simulink library "Driver_Long_Lateral"  (R2025a)
settings: Solver=VariableStepAuto  StartTime=0.0  StopTime=10.0  RelTol=1e-3
undefined symbols (not defined in the file): Driver, Vehicle
libraries: Maneuver_Get_Pose x1
Description:
  | Simscape Vehicle Templates Library
  | 
  | Copyright 2018-2025 The MathWorks, Inc.
settings Model: Creator=smiller  LastModifiedBy=smiller
settings SolverCC: AlgebraicLoopSolver=TrustRegion
settings DataIOCC: ReturnWorkspaceOutputs=off
settings DebuggingCC: UnconnectedInputMsg=warning  UnconnectedOutputMsg=warning  UnconnectedLineMsg=warning  ArithmeticOperatorsInVariantConditions=warning
settings ModelReferenceCC: EnableRefExpFcnMdlSchedulingChecks=on
settings SFSimCC: CustomCodeUndefinedFunction=UseInterfaceOnly
settings RTWCC: GPUComputeCapability=3.5  DLArmComputeVersion=19.05

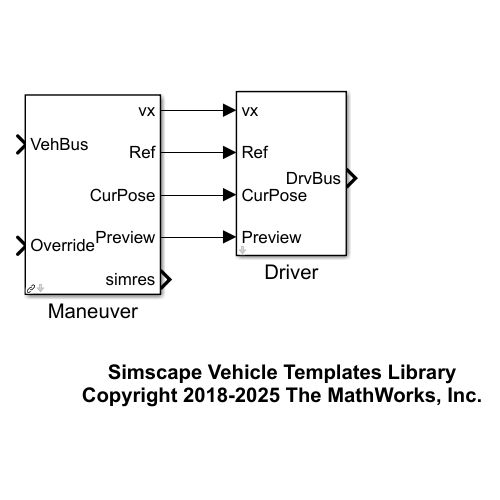
[thumbnail: Simulink's stored preview of the top-level diagram]
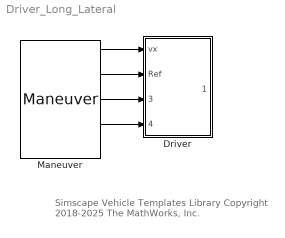
== system Driver_Long_Lateral ==
  note: Simscape Vehicle Templates Library
      | Copyright 2018-2025 The MathWorks, Inc.
  Driver : Subsystem  mask(Driver Behavior){Driver=Driver}
      mask help: Models driver behavior to follow prescribed vehicle trajectory, including path and speed.
  Maneuver : Maneuver_Get_Pose/Maneuver  Maneuver=Maneuver  popup_window=No
  wires:
  Maneuver/1 -> Driver/1(vx)
  Maneuver/2 -> Driver/2(Ref)
  Maneuver/3 -> Driver/3(CurPose)
  Maneuver/4 -> Driver/4(Preview)

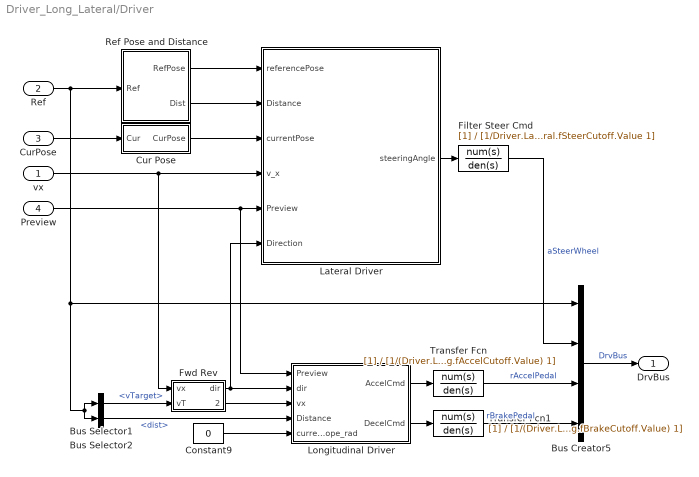
== system Driver_Long_Lateral/Driver ==
  vx : Inport
  Ref : Inport  Port=2
  CurPose : Inport  Port=3
  Preview : Inport  Port=4
  Bus Creator5 : BusCreator  Inputs=4
  Bus Selector1 : BusSelector  OutputSignals=vTarget
  Bus Selector2 : BusSelector  OutputSignals=dist
  Constant9 : Constant  Value=0
  Cur Pose : Subsystem
  Filter Steer Cmd : TransferFcn  Denominator=[1/Driver.Lateral.fSteerCutoff.Value 1]
  Fwd Rev : Subsystem
  Lateral Driver : Subsystem  Variant=on  VariantControlMode=label  VariantControl=Choice  LabelModeActiveChoice=Stanley  mask{Lateral=Driver.Lateral, VariantLabel=Driver.Lateral.class.Value}
      mask prompts: Lateral "Lateral Driver Parameters (structure)"; VariantLabel "Variant Label"
      mask init:
      | curblk = gcb;
      | 
      | % Set variant for this block 
      | set_param(curblk,'LabelModeActiveChoice',VariantLabel);
  Longitudinal Driver : Subsystem  mask(Longitudinal Driver (Velocity-tracking Controller)){SPEED_LOOKAHEAD_TIME=Driver.Long.FFLookahead.Value, C_ROLLING_RESISTANCE_COEFF=Driver.Long.NRollingResistance.Value, ROAD_FRICTION_COEFF=Driver.Long.NRoadFriction.Value, mVehicle=Driver.Long.mVehicle.Value, gGravity=Driver.Long.gGravity.Value, FTractive=Driver.Long.FTractive.Value, KP_SPEED=Driver.Long.Kp.Value, KI_SPEED=Driver.Long.Ki.Value, MAX_ACCEL_MPS2=Driver.Long.gMaxAccel.Value, MAX_DECEL_MPS2=Driver.Long.gMaxDecel.Value, Cdrag=Vehicle.Chassis.Aero.CD.Value, rho_air=Vehicle.Chassis.Aero.rho_air.Value, ARef=Vehicle.Chassis.Aero.ARef.Value}
      mask prompts: SPEED_LOOKAHEAD_TIME "Lookahead time (s)"; C_ROLLING_RESISTANCE_COEFF "Rolling resistance coefficient"; ROAD_FRICTION_COEFF "Road friction coefficient"; mVehicle "Total Vehicle mass (kg)"; gGravity "Gravity (m/s)"; FTractive "Tractive Force (N)"; KP_SPEED "Proportional gain, Kp"; KI_SPEED "Integral gain, Ki"; MAX_ACCEL_MPS2 "Max acceleration (m/s^2, positive number))"; MAX_DECEL_MPS2 "Max deceleration (m/s^2, must be negative)"; Cdrag "Drag coefficient"; rho_air "Density of air (kg/m^3)"; ARef "Frontal Area (m^2)"
      mask help: Implements a PI controller with feedforward for velocity tracking.
      mask DialogControl cont_feedforward Prompt: Feed-Forward Controller parameters
      mask DialogControl cont_feedback Prompt: Feedback Controller parameters
      mask DialogControl cont_drag Prompt: Drag
  Ref Pose and Distance : Subsystem
  Transfer Fcn : TransferFcn  Denominator=[1/(Driver.Long.fAccelCutoff.Value) 1]
  Transfer Fcn1 : TransferFcn  Denominator=[1/(Driver.Long.fBrakeCutoff.Value) 1]
  DrvBus : Outport  VectorParamsAs1DForOutWhenUnconnected=off
  wires:
  Filter Steer Cmd/1 -> Bus Creator5/2  "aSteerWheel"
  Ref Pose and Distance/1(RefPose) -> Lateral Driver/1(referencePose)
  Ref/1 -> Ref Pose and Distance/1(Ref), Bus Selector1/1, Bus Selector2/1, Bus Creator5/1
  Transfer Fcn/1 -> Bus Creator5/3  "rAccelPedal"
  Transfer Fcn1/1 -> Bus Creator5/4  "rBrakePedal"
  Longitudinal Driver/2(DecelCmd) -> Transfer Fcn1/1
  Longitudinal Driver/1(AccelCmd) -> Transfer Fcn/1
  Bus Creator5/1 -> DrvBus/1  "DrvBus"
  Constant9/1 -> Longitudinal Driver/5(current_slope_rad)
  CurPose/1 -> Cur Pose/1(Cur)
  Cur Pose/1(CurPose) -> Lateral Driver/3(currentPose)
  vx/1 -> Lateral Driver/4(v_x), Fwd Rev/1(vx)
  Fwd Rev/1(dir) -> Lateral Driver/6(Direction), Longitudinal Driver/2(dir)
  Lateral Driver/1(steeringAngle) -> Filter Steer Cmd/1
  Preview/1 -> Lateral Driver/5(Preview), Longitudinal Driver/1(Preview)
  Ref Pose and Distance/2(Dist) -> Lateral Driver/2(Distance)
  Bus Selector1/1 -> Fwd Rev/2(vT)  "<vTarget>"
  Fwd Rev/2(vxFwRv) -> Longitudinal Driver/3(vx)
  Bus Selector2/1 -> Longitudinal Driver/4(Distance)  "<dist>"

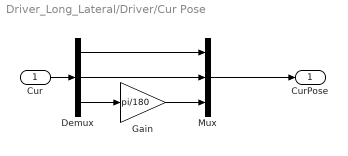
== system Driver_Long_Lateral/Driver/Cur Pose ==
  Cur : Inport
  Demux : Demux  Outputs=3
  Gain : Gain  Gain=pi/180
  Mux : Mux  Inputs=3
  CurPose : Outport  VectorParamsAs1DForOutWhenUnconnected=off
  wires:
  Demux/1 -> Mux/1
  Cur/1 -> Demux/1
  Mux/1 -> CurPose/1
  Demux/2 -> Mux/2
  Demux/3 -> Gain/1
  Gain/1 -> Mux/3

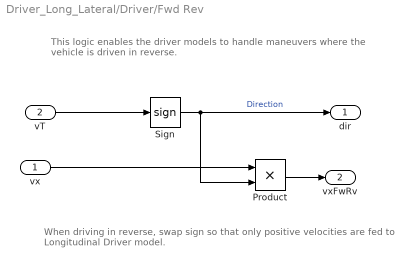
== system Driver_Long_Lateral/Driver/Fwd Rev ==
  note: When driving in reverse, swap sign so that only positive velocities are fed to Longitudinal Driver model.
  note: This logic enables the driver models to handle maneuvers where the vehicle is driven in reverse.
  vx : Inport
  vT : Inport  Port=2
  Product : Product
  Sign : Signum  ZeroCross=off
  dir : Outport
  vxFwRv : Outport  Port=2
  wires:
  vT/1 -> Sign/1
  Sign/1 -> dir/1, Product/2  "Direction"
  vx/1 -> Product/1
  Product/1 -> vxFwRv/1

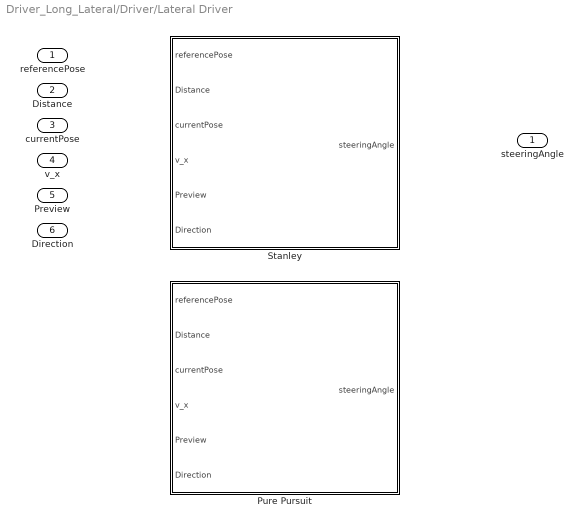
== system Driver_Long_Lateral/Driver/Lateral Driver ==
  referencePose : Inport
  Distance : Inport  Port=2
  currentPose : Inport  Port=3
  v_x : Inport  Port=4
  Preview : Inport  Port=5
  Direction : Inport  Port=6
  Pure Pursuit : Subsystem  VariantControl=Pure_Pursuit  mask(Lateral Driver (Pure Pursuit)){MAX_STEERING_ANGLE_DEG=Lateral.aMaxSteer.Value, L_AXLE_DIST=Lateral.xWheelbase.Value, LOOKAHEAD_GAIN_KPP=Lateral.Pursuit.kLookahead.Value, MIN_LOOKAHEAD_DIST=Lateral.Pursuit.xLookaheadMin.Value, MAX_LOOKAHEAD_DIST=Lateral.Pursuit.xLookaheadMax.Value, HEADING_WEIGHT_KH=Lateral.Pursuit.nWeightHeadingErr.Value}
      mask prompts: MAX_STEERING_ANGLE_DEG "Maximum steering angle (degrees)"; L_AXLE_DIST "Distance from the vehicle's reference point (currentPose) to the front axle (m)"; LOOKAHEAD_GAIN_KPP "Proportional gain for lookahead distance (Ld = K_pp * v_x)"; MIN_LOOKAHEAD_DIST "Minimum lookahead distance (m)"; MAX_LOOKAHEAD_DIST "Maximum lookahead distance (m)"; HEADING_WEIGHT_KH "Weight for the heading error term"
      mask help:
      | Implements PurePursuit method for lateral control.
      | Supports forward and reverse driving.
      | Pure Pursuit is based on Coulter, R. Craig. (1992). Implementation of the Pure Pursuit Path Tracking Algorithm. Carnegie Mellon University, The Robotics Institute. Technical Report CMU-RI-TR-92-01.
      mask DialogControl Container5 Prompt: Vehicle Parameters
      mask DialogControl Container4 Prompt: Pure Pursuit Method Parameters
  Stanley : Subsystem  VariantControl=Stanley  mask(Lateral Driver (Stanley)){MAX_STEERING_ANGLE_DEG=Lateral.aMaxSteer.Value, L_AXLE_DIST=Lateral.xWheelbase.Value, K_cte_forward=Lateral.Stanley.NForward.Value, K_cte_reverse=Lateral.Stanley.NReverse.Value}
      mask prompts: MAX_STEERING_ANGLE_DEG "Maximum steering angle (degrees)"; L_AXLE_DIST "Distance from the vehicle's reference point (currentPose) to the front axle (m)"; K_cte_forward "Cross-track error gain for forward"; K_cte_reverse "Cross-track error gain for reverse"
      mask help:
      | Implements Stanley method for lateral control.
      | Supports forward and reverse driving.
      | Stanley method is based on Hoffmann et al. (2007), "Autonomous Automobile Trajectory Tracking for Off-Road Driving"
      mask DialogControl Container5 Prompt: Vehicle Parameters
      mask DialogControl Container3 Prompt: Stanley Method Parameters
  steeringAngle : Outport

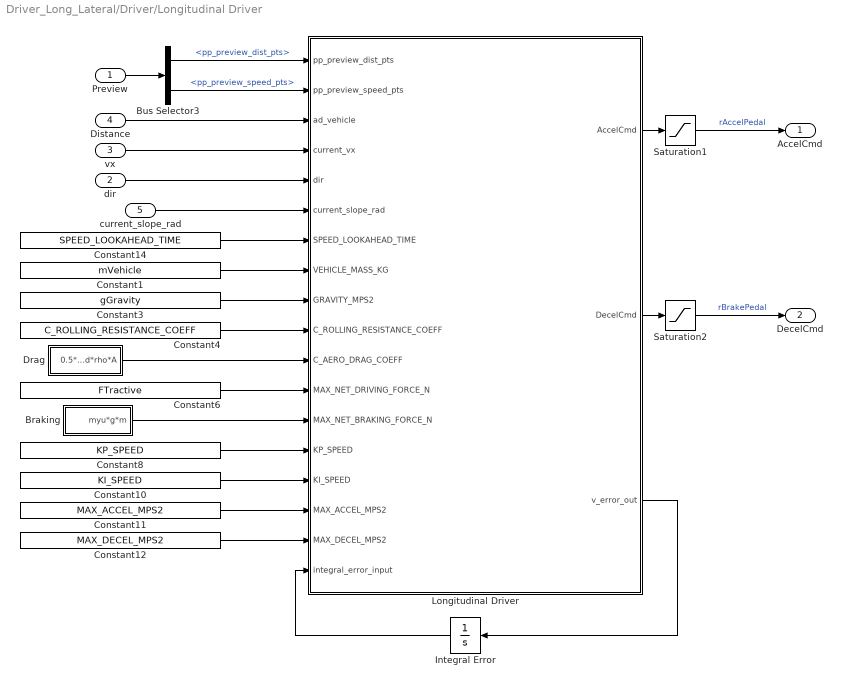
== system Driver_Long_Lateral/Driver/Longitudinal Driver ==
  Preview : Inport
  dir : Inport  Port=2
  vx : Inport  Port=3
  Distance : Inport  Port=4
  current_slope_rad : Inport  Port=5
  Braking : Subsystem
  Bus Selector3 : BusSelector  OutputSignals=pp_preview_dist_pts,pp_preview_speed_pts
  Constant1 : Constant  Value=mVehicle
  Constant10 : Constant  Value=KI_SPEED
  Constant11 : Constant  Value=MAX_ACCEL_MPS2
  Constant12 : Constant  Value=MAX_DECEL_MPS2
  Constant14 : Constant  Value=SPEED_LOOKAHEAD_TIME
  Constant3 : Constant  Value=gGravity
  Constant4 : Constant  Value=C_ROLLING_RESISTANCE_COEFF
  Constant6 : Constant  Value=FTractive
  Constant8 : Constant  Value=KP_SPEED
  Drag : Subsystem
  Integral Error : Integrator
  Longitudinal Driver : MATLAB Function  TreatAsAtomicUnit=on
  Saturation1 : Saturate  UpperLimit=1  LowerLimit=0  ZeroCross=off
  Saturation2 : Saturate  UpperLimit=1  LowerLimit=0  ZeroCross=off
  AccelCmd : Outport
  DecelCmd : Outport  Port=2
  wires:
  Constant6/1 -> Longitudinal Driver/12(MAX_NET_DRIVING_FORCE_N)
  Bus Selector3/1 -> Longitudinal Driver/1(pp_preview_dist_pts)  "<pp_preview_dist_pts>"
  Distance/1 -> Longitudinal Driver/3(ad_vehicle)
  Longitudinal Driver/1(AccelCmd) -> Saturation1/1
  Constant10/1 -> Longitudinal Driver/15(KI_SPEED)
  Constant3/1 -> Longitudinal Driver/9(GRAVITY_MPS2)
  Longitudinal Driver/3(v_error_out) -> Integral Error/1
  Integral Error/1 -> Longitudinal Driver/18(integral_error_input)
  Constant14/1 -> Longitudinal Driver/7(SPEED_LOOKAHEAD_TIME)
  Constant4/1 -> Longitudinal Driver/10(C_ROLLING_RESISTANCE_COEFF)
  Constant1/1 -> Longitudinal Driver/8(VEHICLE_MASS_KG)
  Bus Selector3/2 -> Longitudinal Driver/2(pp_preview_speed_pts)  "<pp_preview_speed_pts>"
  Constant8/1 -> Longitudinal Driver/14(KP_SPEED)
  vx/1 -> Longitudinal Driver/4(current_vx)
  Longitudinal Driver/2(DecelCmd) -> Saturation2/1
  Preview/1 -> Bus Selector3/1
  Saturation1/1 -> AccelCmd/1  "rAccelPedal"
  Saturation2/1 -> DecelCmd/1  "rBrakePedal"
  current_slope_rad/1 -> Longitudinal Driver/6(current_slope_rad)
  Constant11/1 -> Longitudinal Driver/16(MAX_ACCEL_MPS2)
  dir/1 -> Longitudinal Driver/5(dir)
  Constant12/1 -> Longitudinal Driver/17(MAX_DECEL_MPS2)
  Drag/1(0.5*Cd*rho*A) -> Longitudinal Driver/11(C_AERO_DRAG_COEFF)
  Braking/1(myu*g*m) -> Longitudinal Driver/13(MAX_NET_BRAKING_FORCE_N)

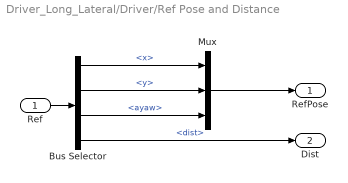
== system Driver_Long_Lateral/Driver/Ref Pose and Distance ==
  Ref : Inport
  Bus Selector : BusSelector  OutputSignals=x,y,ayaw,dist
  Mux : Mux  Inputs=3
  RefPose : Outport  VectorParamsAs1DForOutWhenUnconnected=off
  Dist : Outport  Port=2  VectorParamsAs1DForOutWhenUnconnected=off
  wires:
  Bus Selector/3 -> Mux/3  "<ayaw>"
  Bus Selector/2 -> Mux/2  "<y>"
  Mux/1 -> RefPose/1
  Ref/1 -> Bus Selector/1
  Bus Selector/1 -> Mux/1  "<x>"
  Bus Selector/4 -> Dist/1  "<dist>"

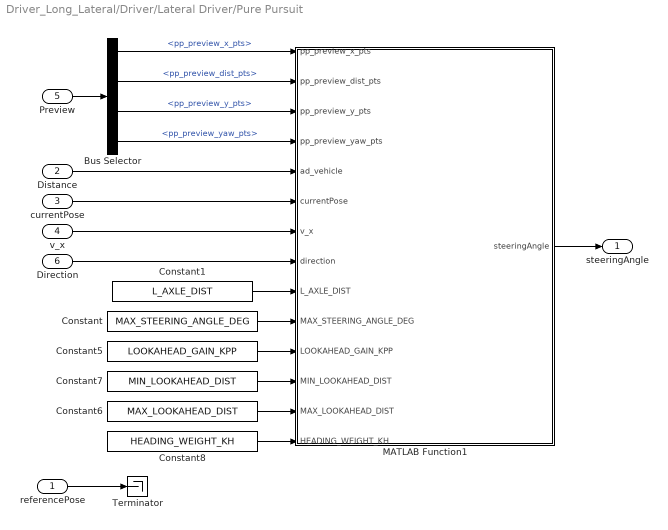
== system Driver_Long_Lateral/Driver/Lateral Driver/Pure Pursuit ==
  referencePose : Inport
  Distance : Inport  Port=2
  currentPose : Inport  Port=3
  v_x : Inport  Port=4
  Preview : Inport  Port=5
  Direction : Inport  Port=6
  Bus Selector : BusSelector  OutputSignals=pp_preview_x_pts,pp_preview_dist_pts,pp_preview_y_pts,pp_preview_yaw_pts
  Constant : Constant  Value=MAX_STEERING_ANGLE_DEG
  Constant1 : Constant  Value=L_AXLE_DIST
  Constant5 : Constant  Value=LOOKAHEAD_GAIN_KPP
  Constant6 : Constant  Value=MAX_LOOKAHEAD_DIST
  Constant7 : Constant  Value=MIN_LOOKAHEAD_DIST
  Constant8 : Constant  Value=HEADING_WEIGHT_KH
  MATLAB Function1 : MATLAB Function  TreatAsAtomicUnit=on
  Terminator : Terminator
  steeringAngle : Outport
  wires:
  Constant8/1 -> MATLAB Function1/14(HEADING_WEIGHT_KH)
  Bus Selector/4 -> MATLAB Function1/4(pp_preview_yaw_pts)  "<pp_preview_yaw_pts>"
  Bus Selector/3 -> MATLAB Function1/3(pp_preview_y_pts)  "<pp_preview_y_pts>"
  Bus Selector/2 -> MATLAB Function1/2(pp_preview_dist_pts)  "<pp_preview_dist_pts>"
  Bus Selector/1 -> MATLAB Function1/1(pp_preview_x_pts)  "<pp_preview_x_pts>"
  Distance/1 -> MATLAB Function1/5(ad_vehicle)
  Preview/1 -> Bus Selector/1
  Constant7/1 -> MATLAB Function1/12(MIN_LOOKAHEAD_DIST)
  Constant6/1 -> MATLAB Function1/13(MAX_LOOKAHEAD_DIST)
  Constant5/1 -> MATLAB Function1/11(LOOKAHEAD_GAIN_KPP)
  MATLAB Function1/1(steeringAngle) -> steeringAngle/1
  Constant1/1 -> MATLAB Function1/9(L_AXLE_DIST)
  Constant/1 -> MATLAB Function1/10(MAX_STEERING_ANGLE_DEG)
  Direction/1 -> MATLAB Function1/8(direction)
  currentPose/1 -> MATLAB Function1/6(currentPose)
  v_x/1 -> MATLAB Function1/7(v_x)
  referencePose/1 -> Terminator/1

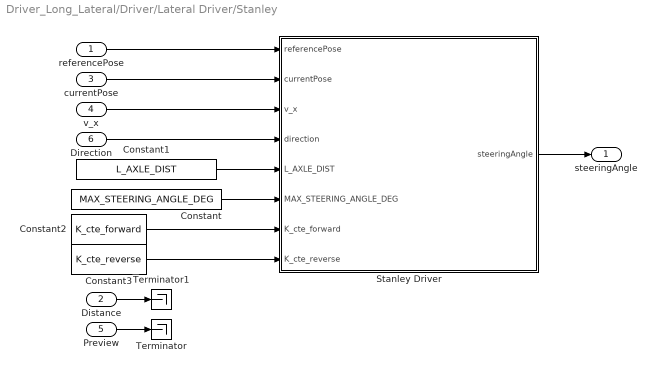
== system Driver_Long_Lateral/Driver/Lateral Driver/Stanley ==
  referencePose : Inport
  Distance : Inport  Port=2
  currentPose : Inport  Port=3
  v_x : Inport  Port=4
  Preview : Inport  Port=5
  Direction : Inport  Port=6
  Constant : Constant  Value=MAX_STEERING_ANGLE_DEG
  Constant1 : Constant  Value=L_AXLE_DIST
  Constant2 : Constant  Value=K_cte_forward
  Constant3 : Constant  Value=K_cte_reverse
  Stanley Driver : MATLAB Function  TreatAsAtomicUnit=on  mask(Lateral Driver (Stanley Driver)){}
      mask help:
      | Implements Stanley method for lateral control.
      | Supports forward and reverse driving.
      | Based on Hoffmann et al. (2007), "Autonomous Automobile Trajectory Tracking for Off-Road Driving"
  Terminator : Terminator
  Terminator1 : Terminator
  steeringAngle : Outport
  wires:
  v_x/1 -> Stanley Driver/3(v_x)
  currentPose/1 -> Stanley Driver/2(currentPose)
  Direction/1 -> Stanley Driver/4(direction)
  referencePose/1 -> Stanley Driver/1(referencePose)
  Constant/1 -> Stanley Driver/6(MAX_STEERING_ANGLE_DEG)
  Constant1/1 -> Stanley Driver/5(L_AXLE_DIST)
  Constant2/1 -> Stanley Driver/7(K_cte_forward)
  Constant3/1 -> Stanley Driver/8(K_cte_reverse)
  Stanley Driver/1(steeringAngle) -> steeringAngle/1
  Preview/1 -> Terminator/1
  Distance/1 -> Terminator1/1

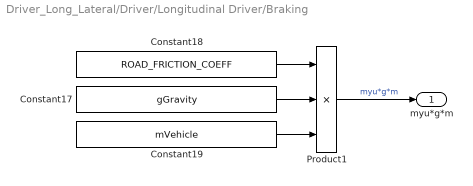
== system Driver_Long_Lateral/Driver/Longitudinal Driver/Braking ==
  Constant17 : Constant  Value=gGravity
  Constant18 : Constant  Value=ROAD_FRICTION_COEFF
  Constant19 : Constant  Value=mVehicle
  Product1 : Product  Inputs=3
  myu*g*m : Outport
  wires:
  Constant17/1 -> Product1/2
  Product1/1 -> myu*g*m/1  "myu*g*m"
  Constant18/1 -> Product1/1
  Constant19/1 -> Product1/3

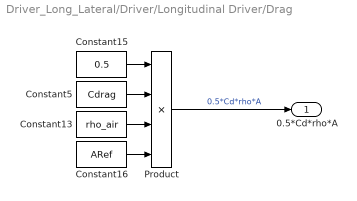
== system Driver_Long_Lateral/Driver/Longitudinal Driver/Drag ==
  Constant13 : Constant  Value=rho_air
  Constant15 : Constant  Value=0.5
  Constant16 : Constant  Value=ARef
  Constant5 : Constant  Value=Cdrag
  Product : Product  Inputs=4
  0.5*Cd*rho*A : Outport
  wires:
  Constant15/1 -> Product/1
  Constant13/1 -> Product/3
  Constant5/1 -> Product/2
  Constant16/1 -> Product/4
  Product/1 -> 0.5*Cd*rho*A/1  "0.5*Cd*rho*A"

== matlab function Driver_Long_Lateral/Driver/Lateral Driver/Stanley/Stanley Driver ==
  data: referencePose input; steeringAngle output; currentPose input; v_x input; direction input; L_AXLE_DIST input; MAX_STEERING_ANGLE_DEG input; K_cte_forward input; K_cte_reverse input
function steeringAngle = lateralDrivingController(referencePose, currentPose, v_x, direction, L_AXLE_DIST, MAX_STEERING_ANGLE_DEG, K_cte_forward, K_cte_reverse)
%#codegen % Directive for MATLAB Coder

% lateralDrivingController Implements Stanley method for lateral control.
% Supports forward and reverse driving.
% Based on Hoffmann et al. (2007), "Autonomous Automobile Trajectory Tracking for Off-Road Driving"
%
% Inputs:
%   referencePose: [x_ref, y_ref, yaw_ref] (1x3 double vector)
%       x_ref: Reference x-coordinate (m) on the path (closest point)
%       y_ref: Reference y-coordinate (m) on the path (closest point)
%       yaw_ref: Reference yaw angle (rad) of the path tangent at (x_ref, y_ref)
%   currentPose: [x_curr, y_curr, yaw_curr] (1x3 double vector)
%       x_curr: Current x-coordinate (m) of the vehicle's reference point (e.g., rear axle center)
%       y_curr: Current y-coordinate (m) of the vehicle's reference point
%       yaw_curr: Current yaw angle (rad) of the vehicle
%   v_x: Current longitudinal velocity (m/s) of the vehicle.
%        Positive for forward, can be negative for reverse (though 'direction' input is primary).
%   direction: Driving direction (+1 for forward, -1 for reverse). (scalar double)
%
% Output:
%   steeringAngle: Calculated steering angle (rad) of the front wheels.
%                  Positive for left turn, negative for right turn.

% --- Controller Parameters (Tunable) ---
% K_cte = Driver.Lateral.NForward.Value  ;  % Cross-track error gain (Stanley gain 'k'). Adjust based on vehicle.
              % Typical values: 0.3 to 1.0. Higher values lead to more aggressive correction.

% L_AXLE_DIST = Driver.Lateral.xWheelbase.Value; % Distance from the vehicle's reference point (currentPose)
                                                % to the front axle (m). If currentPose is rear axle, this is wheelbase.

SOFTENING_CONSTANT_V = 0.1; % Small constant (epsilon) to prevent division by zero or
                            % overly aggressive steering at very low speeds (m/s).
                            % Should be small, e.g., 0.01 to 0.5.

MAX_STEERING_ANGLE = MAX_STEERING_ANGLE_DEG * (pi/180)  ; % Maximum steering angle (radians)
% MIN_VELOCITY_FOR_CONTROL is implicitly handled by SOFTENING_CONSTANT_V and using abs(v_x)

% --- Input Validation / Pre-processing (Basic) ---
referencePose = referencePose(:)';
currentPose = currentPose(:)';

% --- Extract Pose Components ---
x_vehicle_ref_pt   = currentPose(1); % x of vehicle's defined reference point (e.g., rear axle)
y_vehicle_ref_pt   = currentPose(2); % y of vehicle's defined reference point
yaw_vehicle        = currentPose(3); % Vehicle's current yaw angle

x_path   = referencePose(1); % x of closest point on path
y_path   = referencePose(2); % y of closest point on path
yaw_path = referencePose(3); % Tangent angle of path at (x_path, y_path)

% --- 1. Calculate Front Axle Position ---
% Stanley controller operates on the error at the front axle.
% (x_fa, y_fa) in the paper's notation.
x_front_axle = x_vehicle_ref_pt + L_AXLE_DIST * cos(yaw_vehicle);
y_front_axle = y_vehicle_ref_pt + L_AXLE_DIST * sin(yaw_vehicle);

% --- 2. Calculate Heading Error (phi_e in paper, psi_e here) ---
% Difference between path yaw and vehicle yaw.
% phi_e = yaw_path - yaw_vehicle
heading_error_raw = yaw_path - yaw_vehicle;
psi_e = atan2(sin(heading_error_raw), cos(heading_error_raw)); % Normalize to [-pi, pi]

% --- 3. Calculate Cross-Track Error (e_fa) at the Front Axle ---
% As per Hoffmann et al. (2007), e_fa is positive if the path is to the
% RIGHT of the vehicle's front axle.
% e_fa = (x_front_axle - x_path) * sin(yaw_path) - (y_front_axle - y_path) * cos(yaw_path);
%
% Let dx_fa = x_front_axle - x_path
% Let dy_fa = y_front_axle - y_path
% The vector from path point to front axle is [dx_fa, dy_fa].
% The path tangent vector is [cos(yaw_path), sin(yaw_path)].
% The path normal vector pointing to the RIGHT of the path is [sin(yaw_path), -cos(yaw_path)].
% e_fa is the projection of [dx_fa, dy_fa] onto this normal vector.
dx_fa = x_front_axle - x_path;
dy_fa = y_front_axle - y_path;

e_fa = dx_fa * sin(yaw_path) - dy_fa * cos(yaw_path);
% Note on sign:
% If front axle is to the LEFT of path, e_fa will be NEGATIVE.
% If front axle is to the RIGHT of path, e_fa will be POSITIVE.

% --- 4. Calculate Steering Angle Components ---

% Cross-track error steering component (delta_e in paper's combined formula)
% delta_e = arctan(k * e_fa / (v_x + softening_constant))
% Use absolute velocity for the denominator to handle forward/reverse consistently
% and add softening constant.
% The paper's v_x in the denominator implies speed magnitude.
effective_velocity_for_atan = abs(v_x) + SOFTENING_CONSTANT_V;

if direction == 1
    delta_cte = atan2(K_cte_forward *  e_fa, effective_velocity_for_atan);
else % if direction == -1
    delta_cte = atan2(K_cte_reverse * -e_fa, effective_velocity_for_atan);
end

% --- 5. Combine Steering Components (Stanley Law) with Directionality ---
% Standard Stanley Law for forward motion:
% steeringAngleUnsaturated = psi_e + delta_cte;
%
% For REVERSE motion (direction = -1):
% The overall steering command needs to be inverted because the vehicle steers
% from the "rear" effectively.
%   - If heading error (psi_e) is positive (path to the left of vehicle yaw),
%     for forward, steer left. For reverse, to make rear go left, steer front right.
%   - If cross-track error (e_fa negative -> front axle left of path),
%     for forward, delta_cte is negative (steer right). For reverse, to make
%     front axle move right (and thus vehicle move right towards path), steer front left.
%
% So, the entire calculated "forward" steering command is multiplied by 'direction'.
steeringAngleUnsaturated = direction * (psi_e + delta_cte);

% --- 6. Saturate Steering Angle ---
if steeringAngleUnsaturated > MAX_STEERING_ANGLE
    steeringAngle = MAX_STEERING_ANGLE;
elseif steeringAngleUnsaturated < -MAX_STEERING_ANGLE
    steeringAngle = -MAX_STEERING_ANGLE;
else
    steeringAngle = steeringAngleUnsaturated;
end

% --- (Optional) Debugging Outputs ---
% coder.extrinsic('fprintf'); % Allow fprintf for debugging during simulation
% fprintf('Dir: %d, YawVeh: %.2f, YawPath: %.2f, psi_e: %.2f\n', direction, yaw_vehicle, yaw_path, psi_e);
% fprintf('x_fa: %.2f, y_fa: %.2f, e_fa: %.2f\n', x_front_axle, y_front_axle, e_fa);
% fprintf('v_x: %.2f, eff_v: %.2f, delta_cte: %.2f\n', v_x, effective_velocity_for_atan, delta_cte);
% fprintf('UnsatSteer: %.3f, Steering cmd: %.3f\n', steeringAngleUnsaturated, steeringAngle);

end

== matlab function Driver_Long_Lateral/Driver/Longitudinal Driver/Longitudinal Driver ==
  settings: sampleTime=0.1
  data: pp_preview_dist_pts input; AccelCmd output; pp_preview_speed_pts input; ad_vehicle input; current_vx input; dir input; current_slope_rad input; SPEED_LOOKAHEAD_TIME input; VEHICLE_MASS_KG input; GRAVITY_MPS2 input; C_ROLLING_RESISTANCE_COEFF input; C_AERO_DRAG_COEFF input; MAX_NET_DRIVING_FORCE_N input; MAX_NET_BRAKING_FORCE_N input; KP_SPEED input; KI_SPEED input; MAX_ACCEL_MPS2 input; MAX_DECEL_MPS2 input; integral_error_input input; DecelCmd output; v_error_out output
function [AccelCmd, DecelCmd, v_error_out] = longitudinalSpeedController(...
    pp_preview_dist_pts, ...     % Preview segment: cumulative distances (m)
    pp_preview_speed_pts, ...    % Preview segment: target speeds (m/s)
    ad_vehicle, ...              % Current distance of vehicle along path (m)
    current_vx, ...              % Vehicle's current longitudinal velocity (m/s)
    dir, current_slope_rad, ...       % Current road slope/gradient (radians, positive for uphill)    
    SPEED_LOOKAHEAD_TIME, ...    % Lookahead time (s)
    VEHICLE_MASS_KG, ...         % Vehicle mass (kg)
    GRAVITY_MPS2, ...            % Acceleration due to gravity (m/s^2)
    C_ROLLING_RESISTANCE_COEFF, ...    % Rolling resistance coefficient
    C_AERO_DRAG_COEFF, ...             % Aerodynamic drag coefficient (0.5 * rho * A * Cd)
    MAX_NET_DRIVING_FORCE_N, ... % Max net driving force at wheels (engine limit - min resistances)
    MAX_NET_BRAKING_FORCE_N, ... % Max net braking force at wheels (brake limit + engine braking if modeled)
    KP_SPEED, ...                % Proportional gain for speed PI controller (normalized value using max_force_contribution)
    KI_SPEED, ...                % Integral gain for speed PI controller (normalized value using max_force_contribution)
    MAX_ACCEL_MPS2, ...          % Max desired acceleration (for feedforward and limiting)
    MAX_DECEL_MPS2, ...          % Max desired deceleration (negative value, e.g., -5 m/s^2)
    integral_error_input)...     % Externally integrated speed error (m) %#ok<INUSD>

%#codegen

% longitudinalSpeedController Implements a PI controller with feedforward
% for velocity tracking, outputting acceleration/deceleration commands and speed error.
% Designed for continuous-time simulation with external error integration.
%
% Outputs:
%   AccelCmd: Normalized acceleration command [0, 1]
%   DecelCmd: Normalized deceleration command [0, 1] (positive value)
%   v_error_out: Current speed error (v_target - v_actual) (m/s)

%  1. Determine Target Velocity and Desired Acceleration from Preview 
lookahead_dist_for_speed = current_vx * SPEED_LOOKAHEAD_TIME;
target_cumulative_dist_for_speed = ad_vehicle + lookahead_dist_for_speed;

num_preview_pts = length(pp_preview_dist_pts);
v_target_at_lookahead = current_vx; % Default to current speed if no preview

thisSeg = 0;
pp_preview_speed_pts = pp_preview_speed_pts*dir;
if num_preview_pts > 0
    if target_cumulative_dist_for_speed <= pp_preview_dist_pts(1)
        v_target_at_lookahead = pp_preview_speed_pts(1);
    elseif target_cumulative_dist_for_speed >= pp_preview_dist_pts(end)
        v_target_at_lookahead = pp_preview_speed_pts(end);
    else
        % Interpolate to find target speed at lookahead distance
        % (Using existing interpolation logic, could be replaced with interp1)
        for n = 1:(num_preview_pts-1)
            if target_cumulative_dist_for_speed >= pp_preview_dist_pts(n) && ...
               target_cumulative_dist_for_speed < pp_preview_dist_pts(n+1)
                % Ensure denominator is not zero for robust interpolation
                fraction_denom = pp_preview_dist_pts(n+1) - pp_preview_dist_pts(n);
                if fraction_denom > 1e-6 % Avoid division by zero if points are coincident
                    fraction = (target_cumulative_dist_for_speed - pp_preview_dist_pts(n)) / fraction_denom;
                    v_target_at_lookahead = pp_preview_speed_pts(n) + ...
                                       fraction * (pp_preview_speed_pts(n+1) - pp_preview_speed_pts(n));
                else % Points are too close, take the speed of the first point of the pair
                    v_target_at_lookahead = pp_preview_speed_pts(n);
                end
                break; 
            end
            thisSeg = n;
        end
         % Handle case where loop finishes, and target is beyond the last segment start but not caught by pp_preview_dist_pts(end)
         if (thisSeg == (num_preview_pts-1)) && (target_cumulative_dist_for_speed >= pp_preview_dist_pts(end))
            v_target_at_lookahead = pp_preview_speed_pts(end);
         end
    end
end

% Determine desired feedforward acceleration based on a short lookahead on the preview path
idx_current_on_preview = 1;
for n = 1:num_preview_pts
    if ad_vehicle >= pp_preview_dist_pts(n)
        idx_current_on_preview = n;
    else
        break;
    end
end

idx_future_on_preview = idx_current_on_preview;
dist_for_accel_calc = current_vx * 0.1; % Short distance ahead for accel calculation (e.g., 0.2s at current speed)
for n = idx_current_on_preview:num_preview_pts
    if (pp_preview_dist_pts(n) - ad_vehicle) >= dist_for_accel_calc
        idx_future_on_preview = n;
        break;
    end
    if n == num_preview_pts % Reached end of preview
        idx_future_on_preview = num_preview_pts;
    end
end

a_desired_feedforward = 0.0; % Initialize
if idx_future_on_preview > idx_current_on_preview && num_preview_pts > 1
    delta_v = pp_preview_speed_pts(idx_future_on_preview) - pp_preview_speed_pts(idx_current_on_preview);
    delta_d = pp_preview_dist_pts(idx_future_on_preview) - pp_preview_dist_pts(idx_current_on_preview);

    if delta_d > 1e-3 % Ensure segment has some physical length
        v_avg_segment = (pp_preview_speed_pts(idx_future_on_preview) + pp_preview_speed_pts(idx_current_on_preview)) / 2.0;
        
        denominator_v_avg = max(0.1, abs(v_avg_segment)); % Robust denominator for delta_t
        delta_t_segment = delta_d / denominator_v_avg;

        MIN_SEGMENT_TIME_FOR_FF = 1e-3; % Min segment time (s) for a meaningful FF accel calculation
        if delta_t_segment > MIN_SEGMENT_TIME_FOR_FF
            a_desired_feedforward = delta_v / delta_t_segment;
        end
    end
end

if(dir>0)
a_desired_feedforward = max(MAX_DECEL_MPS2, min(a_desired_feedforward, MAX_ACCEL_MPS2)); % Clamp
else
a_desired_feedforward = max(-MAX_ACCEL_MPS2, min(a_desired_feedforward, -MAX_DECEL_MPS2)); % Clamp
end


%  2. Calculate Feedforward Force using Simple Vehicle Model 
F_rolling = C_ROLLING_RESISTANCE_COEFF * VEHICLE_MASS_KG * GRAVITY_MPS2 * cos(current_slope_rad);
F_aero    = C_AERO_DRAG_COEFF * current_vx^2;
F_gravity = VEHICLE_MASS_KG * GRAVITY_MPS2 * sin(current_slope_rad);
F_resist = F_rolling + F_aero + F_gravity;
F_wheels_feedforward = VEHICLE_MASS_KG * a_desired_feedforward - F_resist;

%  3. PI Feedback Controller 
v_error = v_target_at_lookahead - current_vx;
P_term = KP_SPEED * v_error;

% I_term uses externally integrated error
I_term_unclamped = KI_SPEED * integral_error_input;

% Anti-windup: Clamp the force contribution of the I-term
% This assumes integral_error_input is the raw integral.
% The clamping limits the *effect* of very large integrated errors.
max_force_contribution = max(MAX_NET_DRIVING_FORCE_N, MAX_NET_BRAKING_FORCE_N);
I_term = max(-max_force_contribution, min(I_term_unclamped, max_force_contribution));

% Change the PI control to physical values
F_pi_correction = max_force_contribution * (P_term + I_term);

%  4. Combine Feedforward and Feedback 
F_total_desired_at_wheels = F_wheels_feedforward + F_pi_correction;

%  5. Convert Total Desired Force to Normalized Actuation Command [-1, +1] 
actuationCmd = 0.0; % This is the command before any (external) rate limiting

if F_total_desired_at_wheels > 0 % Needs net driving force
    if MAX_NET_DRIVING_FORCE_N > 1e-6 
        actuationCmd = F_total_desired_at_wheels / MAX_NET_DRIVING_FORCE_N;
    end
    actuationCmd = max(0, min(actuationCmd, 1.0)); % Clamp to [0, 1]

elseif F_total_desired_at_wheels < 0 % Needs net braking force
    if MAX_NET_BRAKING_FORCE_N > 1e-6
        actuationCmd = F_total_desired_at_wheels / MAX_NET_BRAKING_FORCE_N; % Will be negative
    end
    actuationCmd = max(-1.0, min(actuationCmd, 0)); % Clamp to [-1, 0]
else
    actuationCmd = 0.0; % Coast
end

% Ensure strictly within [-1, 1] (already handled by clamping in step 5)
% actuationCmd = max(-1.0, min(actuationCmd, 1.0));

% Outputs
if actuationCmd >= 0
    AccelCmd = actuationCmd;
    DecelCmd = 0.0;
else
    AccelCmd = 0.0;
    DecelCmd = -actuationCmd; % DecelCmd is positive, range [0, 1]
end

v_error_out = v_error; % Output current speed error for external integration

%  Debugging Outputs (Optional, ensure coder.extrinsic if used in codegen)
% coder.extrinsic('fprintf');
% fprintf('Vcurr: %.2f, Vtgt_LH: %.2f, Verr: %.2f\n', current_vx, v_target_at_lookahead, v_error);
% fprintf('Ades_FF: %.2f, F_wheels_FF: %.1f, F_PI: %.1f, F_total_des: %.1f\n', ...
%         a_desired_feedforward, F_wheels_feedforward, F_pi_correction, F_total_desired_at_wheels);
% fprintf('CmdUnrated: %.3f\n', actuationCmd);

end

== matlab function Driver_Long_Lateral/Driver/Lateral Driver/Pure Pursuit/MATLAB Function1 ==
  data: pp_preview_x_pts input; pp_preview_dist_pts input; steeringAngle output; pp_preview_y_pts input; pp_preview_yaw_pts input; ad_vehicle input; currentPose input; v_x input; direction input; L_AXLE_DIST input; MAX_STEERING_ANGLE_DEG input; LOOKAHEAD_GAIN_KPP input; MIN_LOOKAHEAD_DIST input; MAX_LOOKAHEAD_DIST input; HEADING_WEIGHT_KH input
function steeringAngle = purePursuitLateralController( ...
    pp_preview_x_pts, pp_preview_dist_pts, pp_preview_y_pts, pp_preview_yaw_pts,  ... % Preview segment
    ad_vehicle,...           % Current distance of vehicle along path (from getPoseCurRef)
    currentPose,...          % Vehicle's current pose: [x_curr, y_curr, yaw_curr_rad]
    v_x,...                  % Vehicle's current longitudinal velocity (m/s)
    direction, ...           % Driving direction: +1 for forward, -1 for reverse
    L_AXLE_DIST, ...         % Wheelbase (m)
    MAX_STEERING_ANGLE_DEG,... % Max steering angle in degrees
    LOOKAHEAD_GAIN_KPP, ...  % Proportional gain for lookahead distance (Ld = K_pp * v_x)
    MIN_LOOKAHEAD_DIST,...   % Minimum lookahead distance (m)
    MAX_LOOKAHEAD_DIST, ...  % Maximum lookahead distance (m)
    HEADING_WEIGHT_KH)       %  Weight for the heading error term 
%#codegen

% purePursuitLateralController Implements Pure Pursuit with dynamic lookahead point selection.
%
% Inputs:
%   pp_preview_x_pts, ..._y_pts, ..._yaw_pts: Arrays of x, y, yaw for path preview segment.
%   pp_preview_dist_pts: Array of cumulative distances for the preview points.
%   ad_vehicle: Current projected cumulative distance of the vehicle along the path.
%   currentPose: [x_vehicle_ref_pt, y_vehicle_ref_pt, yaw_vehicle_rad]
%   v_x: Current longitudinal velocity of the vehicle (m/s).
%   direction: Driving direction (+1 for forward, -1 for reverse).
%   L_AXLE_DIST: Wheelbase (m).
%   MAX_STEERING_ANGLE_DEG: Maximum allowable steering angle (degrees).
%   LOOKAHEAD_GAIN_KPP: Lookahead distance gain (Ld proportional to v_x).
%   MIN_LOOKAHEAD_DIST: Minimum lookahead distance.
%   MAX_LOOKAHEAD_DIST: Maximum lookahead distance.
%   HEADING_WEIGHT_KH:  Weight for the heading error term 
%
% Output:
%   steeringAngle: Calculated steering angle (radians). Positive for left.

%  Parameters 
MAX_STEERING_ANGLE_RAD = MAX_STEERING_ANGLE_DEG * (pi/180);

%  Input Validation / Pre-processing 
% Assuming inputs are already correctly sized (e.g., row vectors for preview points)
currentPose = currentPose(:)'; % Ensure currentPose is a row vector

%  Extract Current Pose Components 
x_vehicle_ref_pt = currentPose(1);
y_vehicle_ref_pt = currentPose(2);
yaw_vehicle_rad  = currentPose(3);

%  1. Calculate Target Lookahead Distance (Ld) 
% Ld is proportional to speed, clamped by min/max values.
% Using abs(v_x) for speed magnitude.
Ld_target = LOOKAHEAD_GAIN_KPP * abs(v_x);
Ld_target = max(MIN_LOOKAHEAD_DIST, min(Ld_target, MAX_LOOKAHEAD_DIST));

%  2. Determine the Actual Lookahead Point on the Preview Segment 
% Target cumulative distance for the lookahead point on the path
target_cumulative_dist_on_path = ad_vehicle + Ld_target;

% Find the point in the preview segment closest to this target_cumulative_dist_on_path
% This assumes pp_preview_dist_pts is sorted (which it is, from linspace).
num_preview_pts = length(pp_preview_dist_pts);
if num_preview_pts == 0
    % Should not happen if getPoseCurRef provides points. Fallback if it does.
    steeringAngle = 0.0;
    % coder.varsize('error_msg'); error('PurePursuit:NoPreviewPoints', 'Preview path is empty.');
    return;
end

min_dist_diff = inf;
idx_lookahead = 1; % Default to the first point

for i = 1:num_preview_pts
    dist_diff = abs(pp_preview_dist_pts(i) - target_cumulative_dist_on_path);
    if dist_diff < min_dist_diff
        min_dist_diff = dist_diff;
        idx_lookahead = i;
    end
end

% Selected lookahead point in global frame
x_lookahead_global = pp_preview_x_pts(idx_lookahead);
y_lookahead_global = pp_preview_y_pts(idx_lookahead);
yaw_path_at_lookahead_rad = pp_preview_yaw_pts(idx_lookahead); % Available if needed

%  3. Transform Lookahead Point to Vehicle's Coordinate Frame 
% Vehicle's reference point (e.g., rear axle) is at the origin of the vehicle frame.
dx_global = x_lookahead_global - x_vehicle_ref_pt;
dy_global = y_lookahead_global - y_vehicle_ref_pt;

cos_yaw_veh = cos(yaw_vehicle_rad);
sin_yaw_veh = sin(yaw_vehicle_rad);

% x_lookahead_vehicle_frame: Positive if lookahead point is ahead of vehicle ref pt
% y_lookahead_vehicle_frame: Positive if lookahead point is to the left of vehicle's longitudinal axis
x_lookahead_vehicle_frame =  dx_global * cos_yaw_veh + dy_global * sin_yaw_veh;
y_lookahead_vehicle_frame = -dx_global * sin_yaw_veh + dy_global * cos_yaw_veh;

%  4. Calculate Curvature (Kappa) 
% Kappa = 2 * y_vehicle_frame / (lookahead_distance_squared)
% Lookahead distance (L_d_actual) is the straight-line distance to the selected point.
L_d_actual_squared = x_lookahead_vehicle_frame^2 + y_lookahead_vehicle_frame^2;

if L_d_actual_squared < 1e-4 % Threshold for small distance squared (e.g., 0.01m dist)
    kappa = 0.0;
else
    kappa = (2 * y_lookahead_vehicle_frame) / L_d_actual_squared;
end

steering_pure_pursuit_term = atan(kappa * L_AXLE_DIST);

%  5. Calculate Heading Error at the Lookahead Point 
% This is the difference between the path's orientation at the lookahead point
% and the vehicle's current orientation.
heading_error_at_lookahead_raw = yaw_path_at_lookahead_rad - yaw_vehicle_rad;
heading_error_at_lookahead = atan2(sin(heading_error_at_lookahead_raw), cos(heading_error_at_lookahead_raw));

%  6. Combine Steering Components 
% steeringAngleUnsaturated_raw = pure_pursuit_term + heading_term_weighted
% The HEADING_WEIGHT_KH determines how much influence the heading error has.
% If KH = 0, it's pure Pure Pursuit.
% If KH > 0, it adds a Stanley-like heading correction.
steeringAngleUnsaturated_raw = steering_pure_pursuit_term + HEADING_WEIGHT_KH * heading_error_at_lookahead;


%  7. Adjust for Driving Direction 
steeringAngleUnsaturated = direction * steeringAngleUnsaturated_raw;

%  8. Saturate Steering Angle 
if steeringAngleUnsaturated > MAX_STEERING_ANGLE_RAD
    steeringAngle = MAX_STEERING_ANGLE_RAD;
elseif steeringAngleUnsaturated < -MAX_STEERING_ANGLE_RAD
    steeringAngle = -MAX_STEERING_ANGLE_RAD;
else
    steeringAngle = steeringAngleUnsaturated;
end

% ... (Optional Debugging) ...
% fprintf('Ld_target: %.2f, Ld_actual_sq: %.2f, PathYawAtLookahead: %.2f\n', Ld_target, L_d_actual_squared, yaw_path_at_lookahead_rad);
% fprintf('PP_term: %.3f, HeadingError: %.3f, HeadingTermWeighted: %.3f\n', steering_pure_pursuit_term, heading_error_at_lookahead, HEADING_WEIGHT_KH * heading_error_at_lookahead);
% fprintf('UnsatRaw: %.3f, SteerCmd: %.3f\n', steeringAngleUnsaturated_raw, steeringAngle);

end
